simulink model "Px4_Attitude"  (R2023b)
settings: Solver=FixedStepAuto  StartTime=0.0  StopTime=500  FixedStep=.02  RelTol=1e-3
values from neighbouring files (symbols this model uses):
  A_Long = [Xu                    Xw                        -w0                            -gravity*cos(theta0) ... (first row only)    [Longitudinal_Autopilot.m]
  B_Long = [Xde                         Xdth ... (first row only)    [Longitudinal_Autopilot.m]
  C_Long = eye(4)    [Longitudinal_Autopilot.m]
  D_Long = zeros(4,2)    [Longitudinal_Autopilot.m]
undefined symbols (not defined in the file or in its folder): gravity, u0, V_tot_0, w0
libraries: simulink_extras x7, slpidlib x3
settings Model: Creator=Saif Mohamed  LastModifiedBy=Saif Mohamed

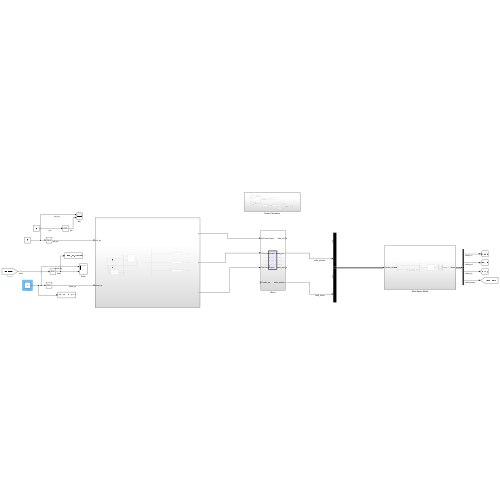
[thumbnail: Simulink's stored preview of the top-level diagram]
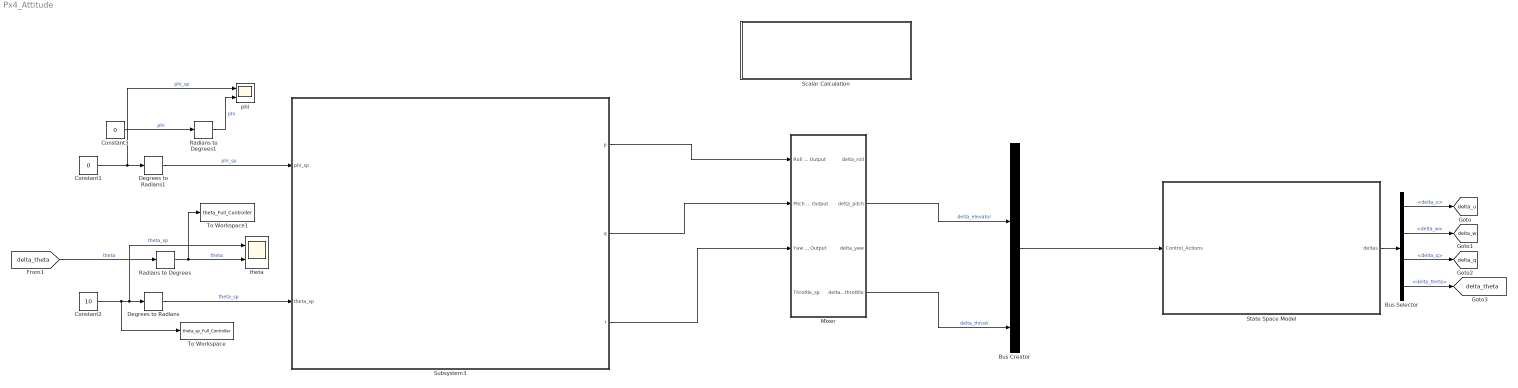
== system Px4_Attitude ==
  Bus Creator : BusCreator  Inputs=4
  Bus Selector : BusSelector  OutputSignals=delta_u,delta_w,delta_q,delta_theta
  Constant1 : Constant  Value=0
  Constant2 : Constant  Value=10
  Constant3 : Constant  Value=0
  Degrees to Radians : simulink_extras/Transformations/Degrees to Radians
  Degrees to Radians1 : simulink_extras/Transformations/Degrees to Radians
  Mixer : Subsystem
  Radians to Degrees : simulink_extras/Transformations/Radians to Degrees
  Radians to Degrees1 : simulink_extras/Transformations/Radians to Degrees
  Scalar Calculation : Subsystem
  State Space Model : Subsystem
  Subsystem3 : Subsystem
  To Workspace : ToWorkspace  VariableName=theta_sp_Full_Controller  SampleTime=-1
  To Workspace1 : ToWorkspace  VariableName=theta_Full_Controller  SampleTime=-1
  phi : Scope  NumInputPorts=2
  theta : Scope  NumInputPorts=2
  tag scope: delta_q=global, delta_theta=global, delta_u=global, delta_w=global
  wires:
  Subsystem3/2(q) -> Mixer/2(Pitch Last Output)
  Radians to Degrees1/1 -> phi/2  "phi"
  Constant1/1 -> phi/1, Degrees to Radians1/1  "phi_sp"
  Constant3/1 -> Radians to Degrees1/1  "phi"
  Subsystem3/3(r) -> Mixer/3(Yaw Last Output)
  Degrees to Radians/1 -> Subsystem3/2(theta_sp)  "theta_sp"
  Radians to Degrees/1 -> To Workspace1/1, theta/2  "theta"
  Mixer/2(delta_pitch) -> Bus Creator/2  "delta_elevator"
  Bus Creator/1 -> State Space Model/1(Control_Actions)
  [delta_theta] -> Radians to Degrees/1  "theta"
  Subsystem3/1(p) -> Mixer/1(Roll Last Output)
  Degrees to Radians1/1 -> Subsystem3/1(phi_sp)  "phi_sp"
  Constant2/1 -> To Workspace/1, theta/1, Degrees to Radians/1  "theta_sp"
  State Space Model/1(deltas) -> Bus Selector/1
  Bus Selector/1 -> [delta_u]  "<delta_u>"
  Bus Selector/2 -> [delta_w]  "<delta_w>"
  Bus Selector/3 -> [delta_q]  "<delta_q>"
  Bus Selector/4 -> [delta_theta]  "<delta_theta>"
  Mixer/4(delta_throttlle) -> Bus Creator/4  "delta_thrust"

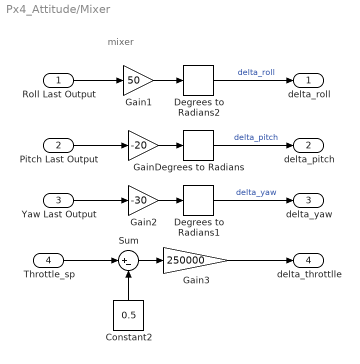
== system Px4_Attitude/Mixer ==
  note: mixer
  Roll Last Output : Inport
  Pitch Last Output : Inport  Port=2
  Yaw Last Output : Inport  Port=3
  Throttle_sp : Inport  Port=4
  Constant2 : Constant  Value=0.5
  Degrees to Radians : simulink_extras/Transformations/Degrees to Radians
  Degrees to Radians1 : simulink_extras/Transformations/Degrees to Radians
  Degrees to Radians2 : simulink_extras/Transformations/Degrees to Radians
  Gain : Gain  Gain=-20
  Gain1 : Gain  Gain=50
  Gain2 : Gain  Gain=-30
  Gain3 : Gain  Gain=250000
  Sum : Sum  Inputs=|+-
  delta_roll : Outport
  delta_pitch : Outport  Port=2
  delta_yaw : Outport  Port=3
  delta_throttlle : Outport  Port=4
  wires:
  Gain2/1 -> Degrees to Radians1/1
  Gain1/1 -> Degrees to Radians2/1
  Degrees to Radians2/1 -> delta_roll/1  "delta_roll"
  Degrees to Radians1/1 -> delta_yaw/1  "delta_yaw"
  Pitch Last Output/1 -> Gain/1
  Degrees to Radians/1 -> delta_pitch/1  "delta_pitch"
  Roll Last Output/1 -> Gain1/1
  Gain/1 -> Degrees to Radians/1
  Yaw Last Output/1 -> Gain2/1
  Constant2/1 -> Sum/2
  Throttle_sp/1 -> Sum/1
  Sum/1 -> Gain3/1
  Gain3/1 -> delta_throttlle/1

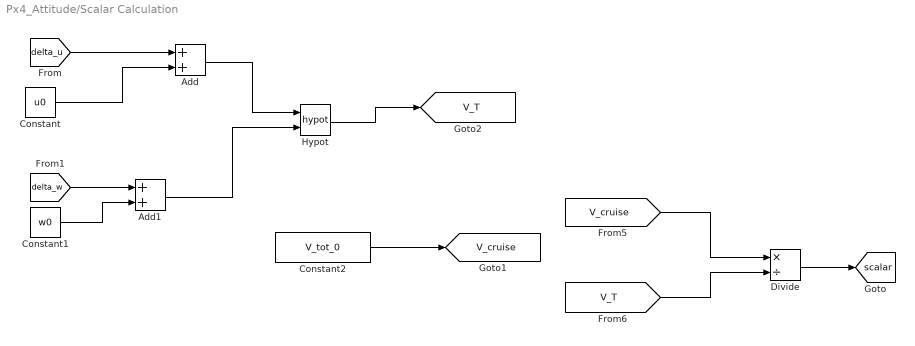
== system Px4_Attitude/Scalar Calculation ==
  Add : Sum
  Add1 : Sum
  Constant : Constant  Value=u0
  Constant1 : Constant  Value=w0
  Constant2 : Constant  Value=V_tot_0
  Divide : Product  Inputs=*/
  Hypot : Math  Operator=hypot
  tag scope: V_T=global, V_cruise=global, scalar=global
  wires:
  [V_T] -> Divide/2
  Constant2/1 -> [V_cruise]
  [V_cruise] -> Divide/1
  Divide/1 -> [scalar]
  Hypot/1 -> [V_T]
  [delta_u] -> Add/1
  Constant/1 -> Add/2
  Add/1 -> Hypot/1
  [delta_w] -> Add1/1
  Constant1/1 -> Add1/2
  Add1/1 -> Hypot/2

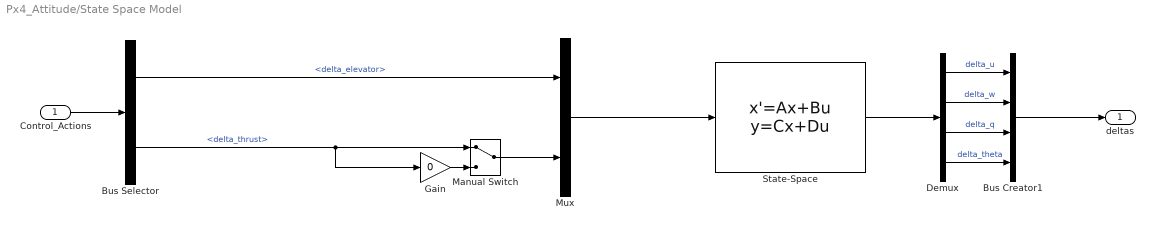
== system Px4_Attitude/State Space Model ==
  Control_Actions : Inport
  Bus Creator1 : BusCreator  Inputs=4
  Bus Selector : BusSelector  OutputSignals=delta_elevator,delta_thrust
  Demux : Demux
  Gain : Gain  Gain=0
  Manual Switch : ManualSwitch
  Mux : Mux  Inputs=2
  State-Space : StateSpace  A=A_Long  B=B_Long  C=C_Long  D=D_Long  InitialCondition=0
  deltas : Outport
  wires:
  Demux/3 -> Bus Creator1/3  "delta_q"
  Mux/1 -> State-Space/1
  Demux/2 -> Bus Creator1/2  "delta_w"
  Demux/1 -> Bus Creator1/1  "delta_u"
  Bus Creator1/1 -> deltas/1
  State-Space/1 -> Demux/1
  Demux/4 -> Bus Creator1/4  "delta_theta"
  Manual Switch/1 -> Mux/2
  Gain/1 -> Manual Switch/2
  Control_Actions/1 -> Bus Selector/1
  Bus Selector/1 -> Mux/1  "<delta_elevator>"
  Bus Selector/2 -> Gain/1, Manual Switch/1  "<delta_thrust>"

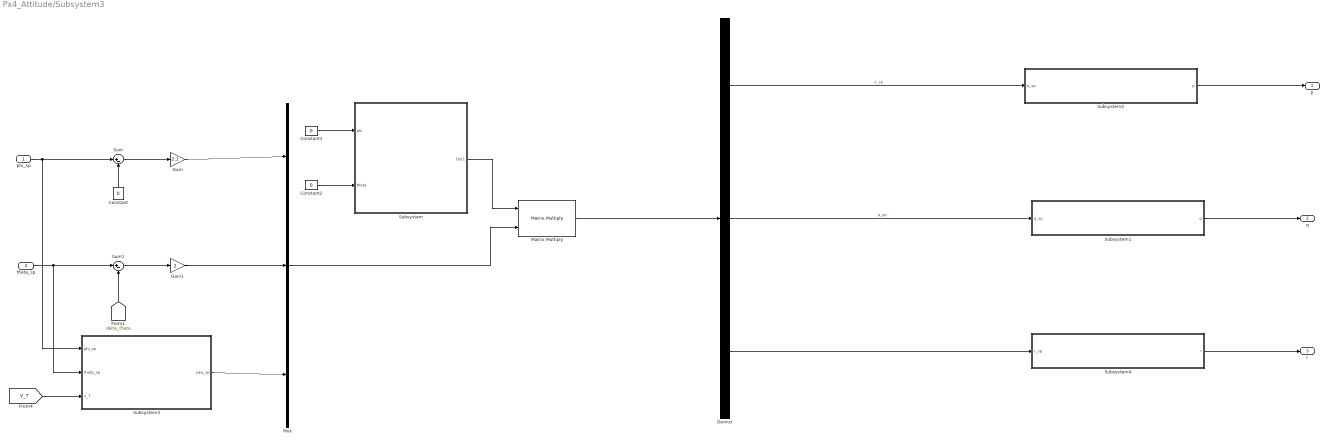
== system Px4_Attitude/Subsystem3 ==
  phi_sp : Inport
  theta_sp : Inport  Port=2
  Constant : Constant  Value=0
  Constant1 : Constant  Value=0
  Constant2 : Constant  Value=0
  Demux : Demux  Outputs=3
  Gain : Gain  Gain=2.1
  Gain1 : Gain  Gain=2
  Matrix Multiply : Product  Multiplication=Matrix(*)
  Mux : Mux  Inputs=3
  Subsystem : Subsystem
  Subsystem1 : Subsystem
  Subsystem2 : Subsystem
  Subsystem3 : Subsystem
  Subsystem4 : Subsystem
  Sum : Sum  Inputs=|+-
  Sum1 : Sum  Inputs=|+-
  p : Outport
  q : Outport  Port=2
  r : Outport  Port=3
  wires:
  Constant/1 -> Sum/2
  phi_sp/1 -> Subsystem3/1(phi_sp), Sum/1
  Sum/1 -> Gain/1
  theta_sp/1 -> Subsystem3/2(theta_sp), Sum1/1
  [delta_theta] -> Sum1/2
  Sum1/1 -> Gain1/1
  Gain/1 -> Mux/1
  Gain1/1 -> Mux/2
  Subsystem/1(Out1) -> Matrix Multiply/1
  Mux/1 -> Matrix Multiply/2
  Matrix Multiply/1 -> Demux/1
  Demux/2 -> Subsystem1/1(q_sp)  "q_sp"
  Demux/1 -> Subsystem2/1(p_sp)  "p_sp"
  Constant1/1 -> Subsystem/1(phi)
  Constant2/1 -> Subsystem/2(theta)
  [V_T] -> Subsystem3/3(v_T)
  Subsystem3/1(yaw_sp) -> Mux/3
  Demux/3 -> Subsystem4/1(r_sp)
  Subsystem2/1(p) -> p/1
  Subsystem1/1(q) -> q/1
  Subsystem4/1(r) -> r/1

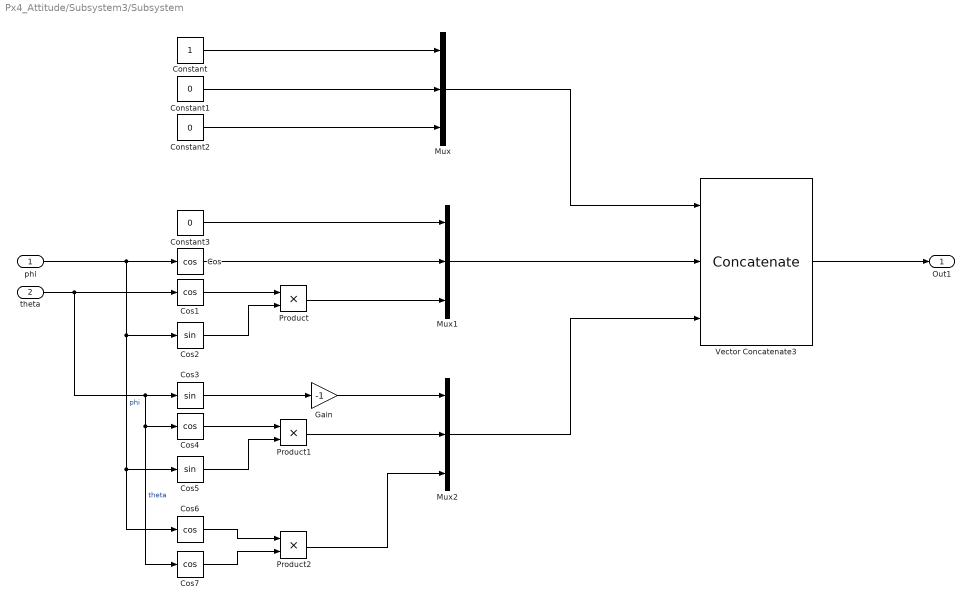
== system Px4_Attitude/Subsystem3/Subsystem ==
  phi : Inport
  theta : Inport  Port=2
  Constant : Constant
  Constant1 : Constant  Value=0
  Constant2 : Constant  Value=0
  Constant3 : Constant  Value=0
  Cos{,1,4,6..7} (5 alike) : Trigonometry  Operator=cos
  Cos2 : Trigonometry
  Cos3 : Trigonometry
  Cos5 : Trigonometry
  Gain : Gain  Gain=-1
  Mux : Mux  Inputs=3
  Mux1 : Mux  Inputs=3
  Mux2 : Mux  Inputs=3
  Product : Product
  Product1 : Product
  Product2 : Product
  Vector Concatenate3 : Concatenate  NumInputs=3  Mode=Multidimensional array  ConcatenateDimension=2
  Out1 : Outport
  wires:
  Constant2/1 -> Mux/3
  Constant1/1 -> Mux/2
  Constant/1 -> Mux/1
  Constant3/1 -> Mux1/1
  Cos/1 -> Mux1/2
  Cos1/1 -> Product/1
  Cos2/1 -> Product/2
  Product/1 -> Mux1/3
  phi/1 -> Cos6/1, Cos5/1, Cos2/1, Cos/1  "phi"
  theta/1 -> Cos7/1, Cos4/1, Cos3/1, Cos1/1  "theta"
  Cos3/1 -> Gain/1
  Gain/1 -> Mux2/1
  Cos5/1 -> Product1/2
  Product1/1 -> Mux2/2
  Cos4/1 -> Product1/1
  Product2/1 -> Mux2/3
  Cos6/1 -> Product2/1
  Cos7/1 -> Product2/2
  Mux2/1 -> Vector Concatenate3/3
  Mux1/1 -> Vector Concatenate3/2
  Mux/1 -> Vector Concatenate3/1
  Vector Concatenate3/1 -> Out1/1

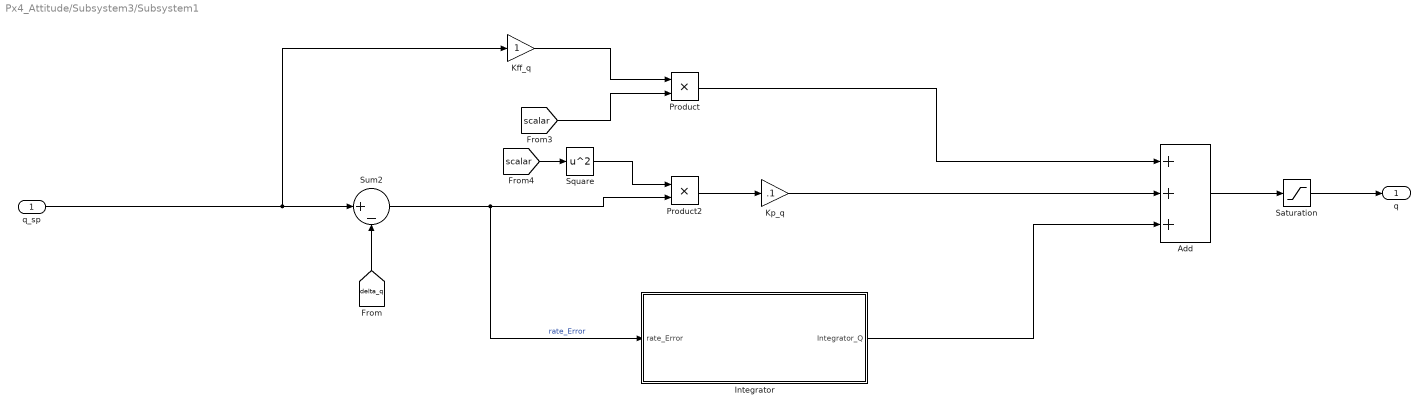
== system Px4_Attitude/Subsystem3/Subsystem1 ==
  q_sp : Inport
  Add : Sum  Inputs=+++
  Integrator : Subsystem
  Kff_q : Gain
  Kp_q : Gain  Gain=.1
  Product : Product
  Product2 : Product
  Saturation : Saturate  UpperLimit=1  LowerLimit=-1
  Square : Math  Operator=square
  Sum2 : Sum  Inputs=|+-
  q : Outport
  wires:
  Kp_q/1 -> Add/2
  [scalar] -> Product/2
  Square/1 -> Product2/1
  [delta_q] -> Sum2/2
  Kff_q/1 -> Product/1
  q_sp/1 -> Kff_q/1, Sum2/1
  Sum2/1 -> Product2/2, Integrator/1(rate_Error)  "rate_Error"
  [scalar] -> Square/1
  Product2/1 -> Kp_q/1
  Product/1 -> Add/1
  Integrator/1(Integrator_Q) -> Add/3
  Add/1 -> Saturation/1
  Saturation/1 -> q/1

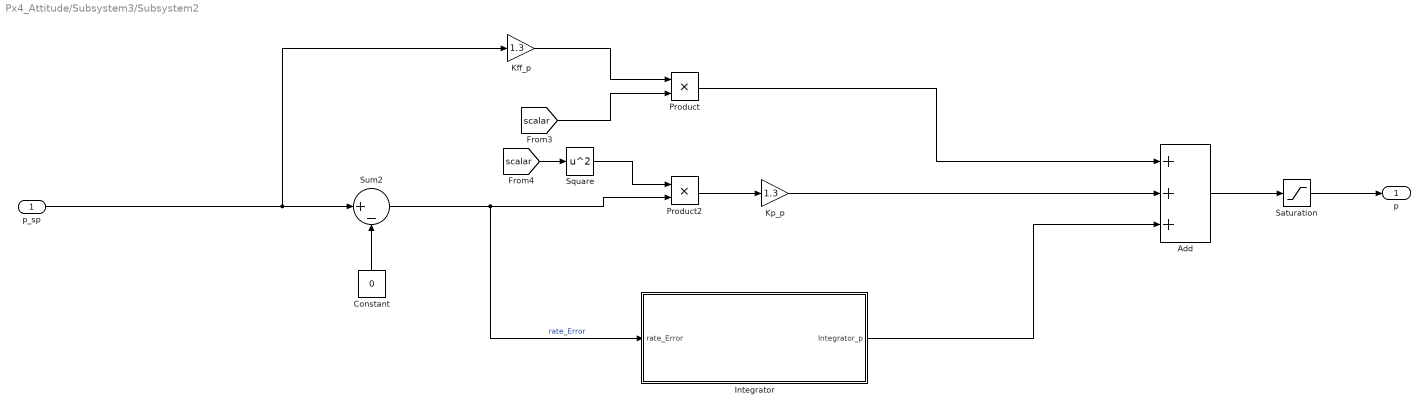
== system Px4_Attitude/Subsystem3/Subsystem2 ==
  p_sp : Inport
  Add : Sum  Inputs=+++
  Constant : Constant  Value=0
  Integrator : Subsystem
  Kff_p : Gain  Gain=1.3
  Kp_p : Gain  Gain=1.3
  Product : Product
  Product2 : Product
  Saturation : Saturate  UpperLimit=1  LowerLimit=-1
  Square : Math  Operator=square
  Sum2 : Sum  Inputs=|+-
  p : Outport
  wires:
  Add/1 -> Saturation/1
  Integrator/1(Integrator_p) -> Add/3
  Product/1 -> Add/1
  Product2/1 -> Kp_p/1
  [scalar] -> Square/1
  Sum2/1 -> Integrator/1(rate_Error), Product2/2  "rate_Error"
  p_sp/1 -> Sum2/1, Kff_p/1
  Kff_p/1 -> Product/1
  Constant/1 -> Sum2/2
  Square/1 -> Product2/1
  [scalar] -> Product/2
  Kp_p/1 -> Add/2
  Saturation/1 -> p/1

== system Px4_Attitude/Subsystem3/Subsystem3 ==
  phi_sp : Inport
  theta_sp : Inport  Port=2
  v_T : Inport  Port=3
  Cos : Trigonometry  Operator=cos
  Divide : Product  Inputs=*/
  Gain : Gain  Gain=gravity
  Product : Product
  Tan : Trigonometry  Operator=tan
  yaw_sp : Outport
  wires:
  phi_sp/1 -> Tan/1
  theta_sp/1 -> Cos/1
  Cos/1 -> Product/2
  Tan/1 -> Product/1
  Product/1 -> Gain/1
  Gain/1 -> Divide/1
  v_T/1 -> Divide/2
  Divide/1 -> yaw_sp/1

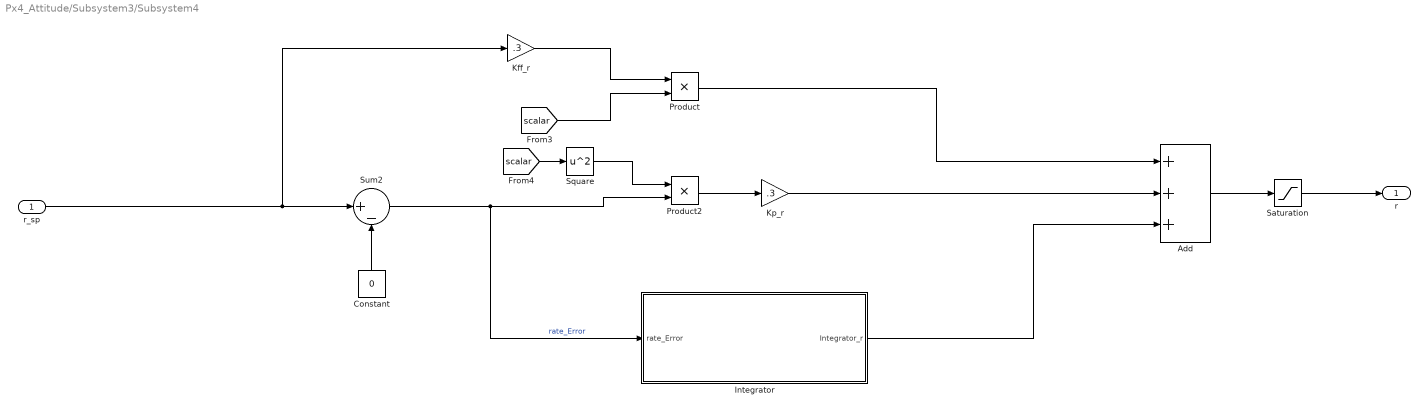
== system Px4_Attitude/Subsystem3/Subsystem4 ==
  r_sp : Inport
  Add : Sum  Inputs=+++
  Constant : Constant  Value=0
  Integrator : Subsystem
  Kff_r : Gain  Gain=.3
  Kp_r : Gain  Gain=.3
  Product : Product
  Product2 : Product
  Saturation : Saturate  UpperLimit=1  LowerLimit=-1
  Square : Math  Operator=square
  Sum2 : Sum  Inputs=|+-
  r : Outport
  wires:
  Add/1 -> Saturation/1
  Integrator/1(Integrator_r) -> Add/3
  Product/1 -> Add/1
  Product2/1 -> Kp_r/1
  [scalar] -> Square/1
  Sum2/1 -> Integrator/1(rate_Error), Product2/2  "rate_Error"
  r_sp/1 -> Sum2/1, Kff_r/1
  Kff_r/1 -> Product/1
  Constant/1 -> Sum2/2
  Square/1 -> Product2/1
  [scalar] -> Product/2
  Kp_r/1 -> Add/2
  Saturation/1 -> r/1

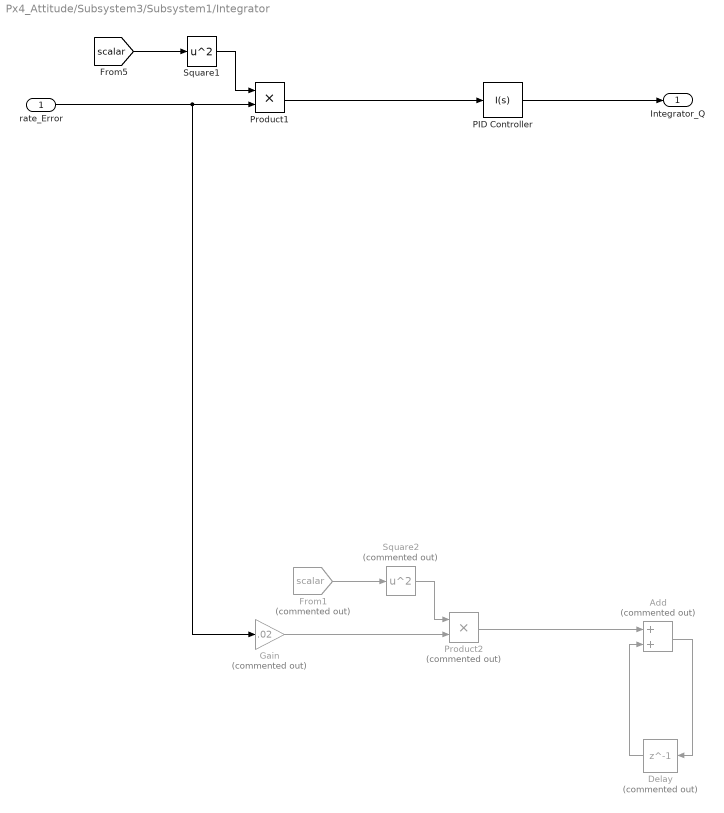
== system Px4_Attitude/Subsystem3/Subsystem1/Integrator ==
  rate_Error : Inport
  Add : Sum  Commented=on
  Delay : Delay  Commented=on  DelayLength=1
  From1 : From  Commented=on  GotoTag=scalar  TagVisibility=global
  Gain : Gain  Commented=on  Gain=.02
  PID Controller : slpidlib/PID Controller  Controller=I  Form=Parallel  TimeDomain=Continuous-time  UseExternalTs=off  SampleTime=-1  IntegratorMethod=Forward Euler  FilterMethod=Forward Euler  ControllerParametersSource=internal  P=1  I=.4  UseKiTs=off  D=0  N=100  UseFilter=on  TunerSelectOption=Transfer Function Based (PID Tuner App)  InitialConditionSource=internal  InitialConditionForIntegrator=0  InitialConditionForFilter=0  DifferentiatorICPrevScaledInput=0  ExternalReset=none  TrackingMode=off  Kt=1  LimitOutput=off  SatLimitsSource=internal  UpperSaturationLimit=inf  LowerSaturationLimit=-inf  LinearizeAsGain=on  AntiWindupMode=none  Kb=1  LimitIntegrator=off  UpperIntegratorSaturationLimit=inf  LowerIntegratorSaturationLimit=-inf  POutMin=[]  POutMax=[]  IOutMin=[]  IOutMax=[]  DOutMin=[]  DOutMax=[]  NOutMin=[]  NOutMax=[]  SumOutMin=[]  SumOutMax=[]  SaturationOutMin=[]  SaturationOutMax=[]  PParamMin=[]  PParamMax=[]  IParamMin=[]  IParamMax=[]  DParamMin=[]  DParamMax=[]  NParamMin=[]  NParamMax=[]  KbParamMin=[]  KbParamMax=[]  KtParamMin=[]  KtParamMax=[]  KbOutMin=[]  KbOutMax=[]  KtOutMin=[]  KtOutMax=[]  IntegratorOutMin=[]  IntegratorOutMax=[]  FilterOutMin=[]  FilterOutMax=[]  SumI1OutMin=[]  SumI1OutMax=[]  SumI2OutMin=[]  SumI2OutMax=[]  SumI3OutMin=[]  SumI3OutMax=[]  SumI4OutMin=[]  SumI4OutMax=[]  SumDOutMin=[]  SumDOutMax=[]  DifferentiatorOutMin=[]  DifferentiatorOutMax=[]  FilterDiffOutCoefMin=[]  FilterDiffOutCoefMax=[]  ReciprocalOutMin=[]  ReciprocalOutMax=[]  SumDenOutMin=[]  SumDenOutMax=[]  SumNumOutMin=[]  SumNumOutMax=[]  DivideOutMin=[]  DivideOutMax=[]  UdiffTsProdOutMin=[]  UdiffTsProdOutMax=[]  NTsProdOutMin=[]  NTsProdOutMax=[]  UintegralTsProdOutMin=[]  UintegralTsProdOutMax=[]  UngainTsProdOutMin=[]  UngainTsProdOutMax=[]  ClampingZeroOutDataTypeStr=Inherit: Inherit via back propagation  ClampingZeroOutMin=[]  ClampingZeroOutMax=[]  FilterDenConstantOutDataTypeStr=Inherit: Inherit via back propagation  FilterDenConstantOutMin=[]  FilterDenConstantOutMax=[]  PCopyOutDataTypeStr=Inherit: Inherit via back propagation  PCopyOutMin=[]  PCopyOutMax=[]  NCopyOutDataTypeStr=Inherit: Inherit via back propagation  NCopyOutMin=[]  NCopyOutMax=[]  IntegratorContinuousStateAttributes=''  IntegratorStateMustResolveToSignalObject=off  IntegratorRTWStateStorageClass=Auto  FilterContinuousStateAttributes=''  FilterStateMustResolveToSignalObject=off  FilterRTWStateStorageClass=Auto  ParallelPVariant=Disabled  IdealPVariant=Disabled  IVariant=InternalParameters  DVariant=Disabled  IntegratorVariant=Continuous  SatVariant=Disabled  AWVariant=Passthrough  PCopyVariant=Disabled  TRVariant=Disabled  FdbkBlocksVariant=Forward  IdealPFdbkVariant=Disabled  SatFdbkVariant=Disabled  DerivativeFilterVariant=Disabled  NVariant=Disabled  NCopyVariant=Disabled_SignalSpec  FilterICVariant=Disabled  IntegratorICVariant=InternalICs  ExternalResetVariant=Disabled  TRSumVariant=Passthrough  SumFdbkVariant=Disabled  SumVariant=Passthrough_I  TsampFilterVariant=InternalTs  TsampNgainVariant=Passthrough  TsampIntegralVariant=Disabled_SignalSpec  ExternalSaturationOutDataTypeStr=Inherit: Same as second input
  Product1 : Product
  Product2 : Product  Commented=on
  Square1 : Math  Operator=square
  Square2 : Math  Commented=on  Operator=square
  Integrator_Q : Outport
  wires:
  [scalar] -> Square1/1
  Product1/1 -> PID Controller/1
  Square1/1 -> Product1/1
  rate_Error/1 -> Gain/1, Product1/2
  Gain/1 -> Product2/2
  Square2/1 -> Product2/1
  From1/1 -> Square2/1
  Product2/1 -> Add/1
  Add/1 -> Delay/1
  Delay/1 -> Add/2
  PID Controller/1 -> Integrator_Q/1

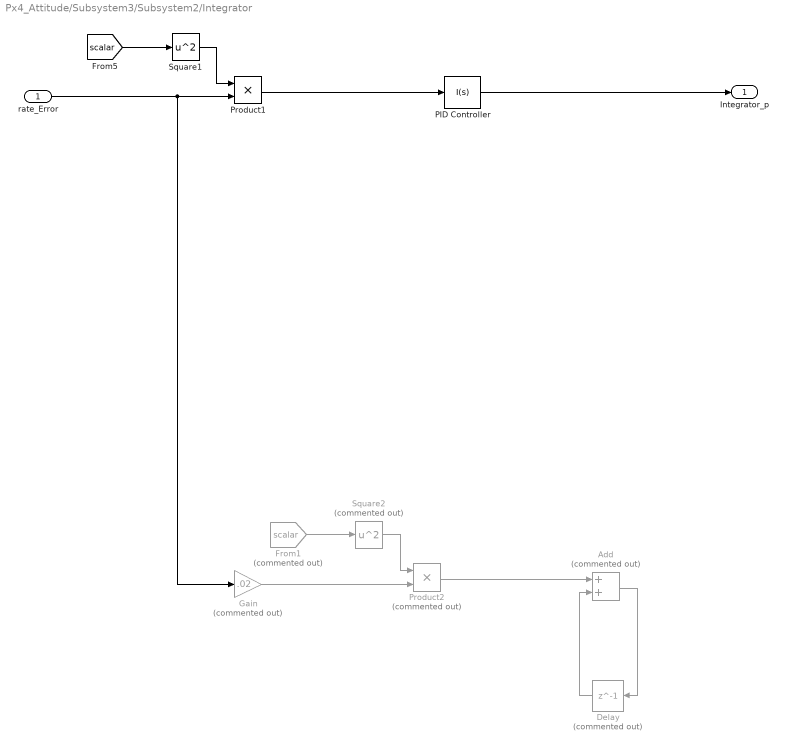
== system Px4_Attitude/Subsystem3/Subsystem2/Integrator ==
  rate_Error : Inport
  Add : Sum  Commented=on
  Delay : Delay  Commented=on  DelayLength=1
  From1 : From  Commented=on  GotoTag=scalar  TagVisibility=global
  Gain : Gain  Commented=on  Gain=.02
  PID Controller : slpidlib/PID Controller  Controller=I  Form=Parallel  TimeDomain=Continuous-time  UseExternalTs=off  SampleTime=-1  IntegratorMethod=Forward Euler  FilterMethod=Forward Euler  ControllerParametersSource=internal  P=1  I=0.085  UseKiTs=off  D=0  N=100  UseFilter=on  TunerSelectOption=Transfer Function Based (PID Tuner App)  InitialConditionSource=internal  InitialConditionForIntegrator=0  InitialConditionForFilter=0  DifferentiatorICPrevScaledInput=0  ExternalReset=none  TrackingMode=off  Kt=1  LimitOutput=off  SatLimitsSource=internal  UpperSaturationLimit=inf  LowerSaturationLimit=-inf  LinearizeAsGain=on  AntiWindupMode=none  Kb=1  LimitIntegrator=off  UpperIntegratorSaturationLimit=inf  LowerIntegratorSaturationLimit=-inf  POutMin=[]  POutMax=[]  IOutMin=[]  IOutMax=[]  DOutMin=[]  DOutMax=[]  NOutMin=[]  NOutMax=[]  SumOutMin=[]  SumOutMax=[]  SaturationOutMin=[]  SaturationOutMax=[]  PParamMin=[]  PParamMax=[]  IParamMin=[]  IParamMax=[]  DParamMin=[]  DParamMax=[]  NParamMin=[]  NParamMax=[]  KbParamMin=[]  KbParamMax=[]  KtParamMin=[]  KtParamMax=[]  KbOutMin=[]  KbOutMax=[]  KtOutMin=[]  KtOutMax=[]  IntegratorOutMin=[]  IntegratorOutMax=[]  FilterOutMin=[]  FilterOutMax=[]  SumI1OutMin=[]  SumI1OutMax=[]  SumI2OutMin=[]  SumI2OutMax=[]  SumI3OutMin=[]  SumI3OutMax=[]  SumI4OutMin=[]  SumI4OutMax=[]  SumDOutMin=[]  SumDOutMax=[]  DifferentiatorOutMin=[]  DifferentiatorOutMax=[]  FilterDiffOutCoefMin=[]  FilterDiffOutCoefMax=[]  ReciprocalOutMin=[]  ReciprocalOutMax=[]  SumDenOutMin=[]  SumDenOutMax=[]  SumNumOutMin=[]  SumNumOutMax=[]  DivideOutMin=[]  DivideOutMax=[]  UdiffTsProdOutMin=[]  UdiffTsProdOutMax=[]  NTsProdOutMin=[]  NTsProdOutMax=[]  UintegralTsProdOutMin=[]  UintegralTsProdOutMax=[]  UngainTsProdOutMin=[]  UngainTsProdOutMax=[]  ClampingZeroOutDataTypeStr=Inherit: Inherit via back propagation  ClampingZeroOutMin=[]  ClampingZeroOutMax=[]  FilterDenConstantOutDataTypeStr=Inherit: Inherit via back propagation  FilterDenConstantOutMin=[]  FilterDenConstantOutMax=[]  PCopyOutDataTypeStr=Inherit: Inherit via back propagation  PCopyOutMin=[]  PCopyOutMax=[]  NCopyOutDataTypeStr=Inherit: Inherit via back propagation  NCopyOutMin=[]  NCopyOutMax=[]  IntegratorContinuousStateAttributes=''  IntegratorStateMustResolveToSignalObject=off  IntegratorRTWStateStorageClass=Auto  FilterContinuousStateAttributes=''  FilterStateMustResolveToSignalObject=off  FilterRTWStateStorageClass=Auto  ParallelPVariant=Disabled  IdealPVariant=Disabled  IVariant=InternalParameters  DVariant=Disabled  IntegratorVariant=Continuous  SatVariant=Disabled  AWVariant=Passthrough  PCopyVariant=Disabled  TRVariant=Disabled  FdbkBlocksVariant=Forward  IdealPFdbkVariant=Disabled  SatFdbkVariant=Disabled  DerivativeFilterVariant=Disabled  NVariant=Disabled  NCopyVariant=Disabled_SignalSpec  FilterICVariant=Disabled  IntegratorICVariant=InternalICs  ExternalResetVariant=Disabled  TRSumVariant=Passthrough  SumFdbkVariant=Disabled  SumVariant=Passthrough_I  TsampFilterVariant=InternalTs  TsampNgainVariant=Passthrough  TsampIntegralVariant=Disabled_SignalSpec  ExternalSaturationOutDataTypeStr=Inherit: Same as second input
  Product1 : Product
  Product2 : Product  Commented=on
  Square1 : Math  Operator=square
  Square2 : Math  Commented=on  Operator=square
  Integrator_p : Outport
  wires:
  Delay/1 -> Add/2
  Add/1 -> Delay/1
  Product2/1 -> Add/1
  From1/1 -> Square2/1
  Square2/1 -> Product2/1
  Gain/1 -> Product2/2
  rate_Error/1 -> Product1/2, Gain/1
  Square1/1 -> Product1/1
  Product1/1 -> PID Controller/1
  [scalar] -> Square1/1
  PID Controller/1 -> Integrator_p/1

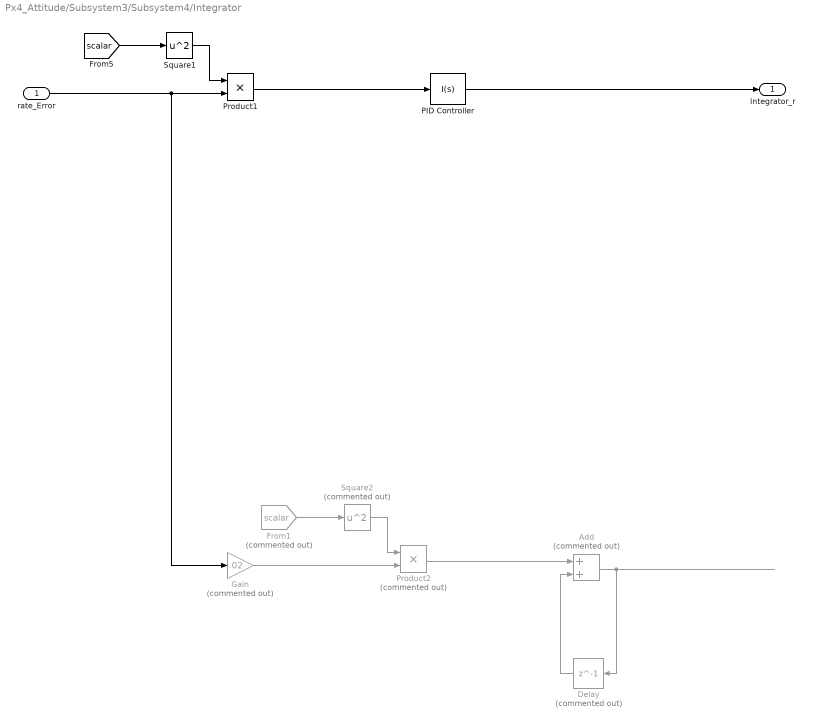
== system Px4_Attitude/Subsystem3/Subsystem4/Integrator ==
  rate_Error : Inport
  Add : Sum  Commented=on
  Delay : Delay  Commented=on  DelayLength=1
  From1 : From  Commented=on  GotoTag=scalar
  Gain : Gain  Commented=on  Gain=.02
  PID Controller : slpidlib/PID Controller  Controller=I  Form=Parallel  TimeDomain=Continuous-time  UseExternalTs=off  SampleTime=-1  IntegratorMethod=Forward Euler  FilterMethod=Forward Euler  ControllerParametersSource=internal  P=1  I=.05  UseKiTs=off  D=0  N=100  UseFilter=on  TunerSelectOption=Transfer Function Based (PID Tuner App)  InitialConditionSource=internal  InitialConditionForIntegrator=0  InitialConditionForFilter=0  DifferentiatorICPrevScaledInput=0  ExternalReset=none  TrackingMode=off  Kt=1  LimitOutput=off  SatLimitsSource=internal  UpperSaturationLimit=inf  LowerSaturationLimit=-inf  LinearizeAsGain=on  AntiWindupMode=none  Kb=1  LimitIntegrator=off  UpperIntegratorSaturationLimit=inf  LowerIntegratorSaturationLimit=-inf  POutMin=[]  POutMax=[]  IOutMin=[]  IOutMax=[]  DOutMin=[]  DOutMax=[]  NOutMin=[]  NOutMax=[]  SumOutMin=[]  SumOutMax=[]  SaturationOutMin=[]  SaturationOutMax=[]  PParamMin=[]  PParamMax=[]  IParamMin=[]  IParamMax=[]  DParamMin=[]  DParamMax=[]  NParamMin=[]  NParamMax=[]  KbParamMin=[]  KbParamMax=[]  KtParamMin=[]  KtParamMax=[]  KbOutMin=[]  KbOutMax=[]  KtOutMin=[]  KtOutMax=[]  IntegratorOutMin=[]  IntegratorOutMax=[]  FilterOutMin=[]  FilterOutMax=[]  SumI1OutMin=[]  SumI1OutMax=[]  SumI2OutMin=[]  SumI2OutMax=[]  SumI3OutMin=[]  SumI3OutMax=[]  SumI4OutMin=[]  SumI4OutMax=[]  SumDOutMin=[]  SumDOutMax=[]  DifferentiatorOutMin=[]  DifferentiatorOutMax=[]  FilterDiffOutCoefMin=[]  FilterDiffOutCoefMax=[]  ReciprocalOutMin=[]  ReciprocalOutMax=[]  SumDenOutMin=[]  SumDenOutMax=[]  SumNumOutMin=[]  SumNumOutMax=[]  DivideOutMin=[]  DivideOutMax=[]  UdiffTsProdOutMin=[]  UdiffTsProdOutMax=[]  NTsProdOutMin=[]  NTsProdOutMax=[]  UintegralTsProdOutMin=[]  UintegralTsProdOutMax=[]  UngainTsProdOutMin=[]  UngainTsProdOutMax=[]  ClampingZeroOutDataTypeStr=Inherit: Inherit via back propagation  ClampingZeroOutMin=[]  ClampingZeroOutMax=[]  FilterDenConstantOutDataTypeStr=Inherit: Inherit via back propagation  FilterDenConstantOutMin=[]  FilterDenConstantOutMax=[]  PCopyOutDataTypeStr=Inherit: Inherit via back propagation  PCopyOutMin=[]  PCopyOutMax=[]  NCopyOutDataTypeStr=Inherit: Inherit via back propagation  NCopyOutMin=[]  NCopyOutMax=[]  IntegratorContinuousStateAttributes=''  IntegratorStateMustResolveToSignalObject=off  IntegratorRTWStateStorageClass=Auto  FilterContinuousStateAttributes=''  FilterStateMustResolveToSignalObject=off  FilterRTWStateStorageClass=Auto  ParallelPVariant=Disabled  IdealPVariant=Disabled  IVariant=InternalParameters  DVariant=Disabled  IntegratorVariant=Continuous  SatVariant=Disabled  AWVariant=Passthrough  PCopyVariant=Disabled  TRVariant=Disabled  FdbkBlocksVariant=Forward  IdealPFdbkVariant=Disabled  SatFdbkVariant=Disabled  DerivativeFilterVariant=Disabled  NVariant=Disabled  NCopyVariant=Disabled_SignalSpec  FilterICVariant=Disabled  IntegratorICVariant=InternalICs  ExternalResetVariant=Disabled  TRSumVariant=Passthrough  SumFdbkVariant=Disabled  SumVariant=Passthrough_I  TsampFilterVariant=InternalTs  TsampNgainVariant=Passthrough  TsampIntegralVariant=Disabled_SignalSpec  ExternalSaturationOutDataTypeStr=Inherit: Same as second input
  Product1 : Product
  Product2 : Product  Commented=on
  Square1 : Math  Operator=square
  Square2 : Math  Commented=on  Operator=square
  Integrator_r : Outport
  wires:
  Delay/1 -> Add/2
  Add/1 -> Delay/1
  Product2/1 -> Add/1
  From1/1 -> Square2/1
  Square2/1 -> Product2/1
  Gain/1 -> Product2/2
  rate_Error/1 -> Product1/2, Gain/1
  Square1/1 -> Product1/1
  Product1/1 -> PID Controller/1
  [scalar] -> Square1/1
  PID Controller/1 -> Integrator_r/1
